simulink model "Non_linear_damper"  (R2023b)
settings: Solver=VariableStepAuto  StartTime=0.0  StopTime=10.0  RelTol=1e-3
values from neighbouring files (symbols this model uses):
  Ks = params.Ks    [Non-_inear_damper.m]    (also in Non_linear_damper.m; Non_linear_damper_v2.m; Sim1_stable.m = 100; Simulation1.m = 100)
  Kt = params.Kt    [Non-_inear_damper.m]    (also in Non_linear_damper.m; Non_linear_damper_v2.m; Sim1_stable.m = 1000; Simulation1.m = 1000)
  ms = params.ms    [Non-_inear_damper.m]    (also in Non_linear_damper.m; Non_linear_damper_v2.m; Sim1_stable.m = 2.59027094234; Simulation1.m = 2.59027094234)
  mu = params.mu    [Non-_inear_damper.m]    (also in Non_linear_damper.m; Non_linear_damper_v2.m; Sim1_stable.m = 0.259027094234; Simulation1.m = 0.259027094234)
settings Model: Creator=youbotica  LastModifiedBy=youbotica

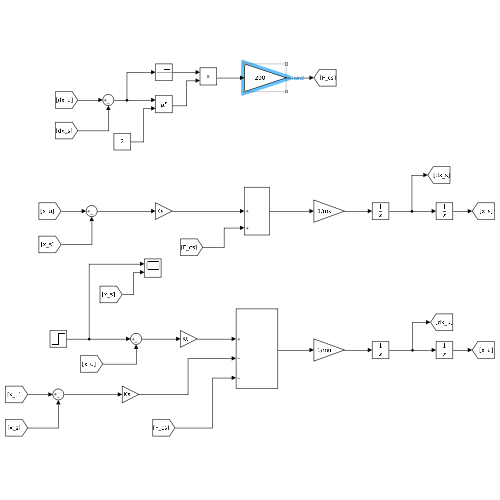
[thumbnail: Simulink's stored preview of the top-level diagram]
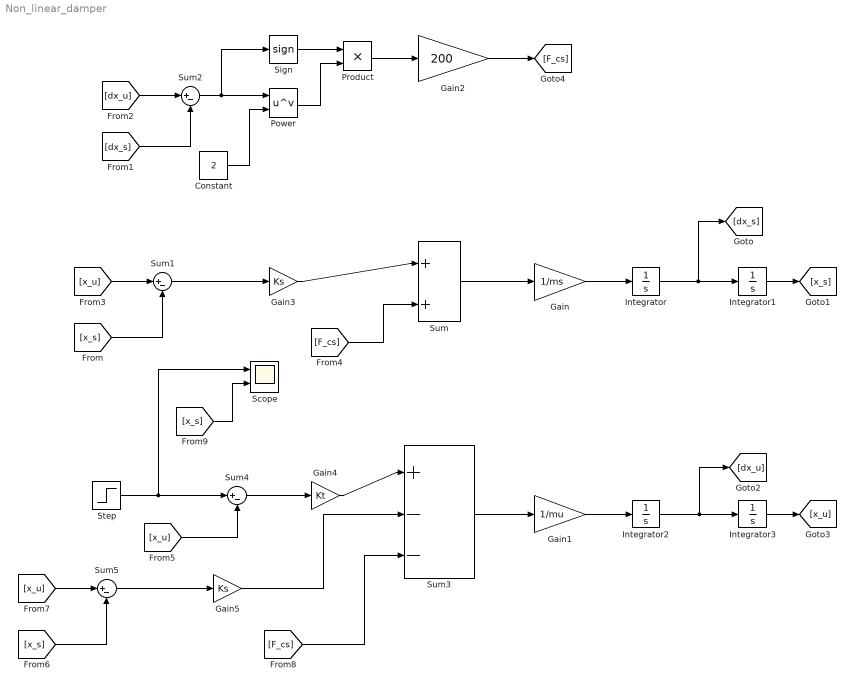
== system Non_linear_damper ==
  Constant : Constant  Value=2
  Gain : Gain  Gain=1/ms
  Gain1 : Gain  Gain=1/mu
  Gain2 : Gain  Gain=200
  Gain3 : Gain  Gain=Ks
  Gain4 : Gain  Gain=Kt
  Gain5 : Gain  Gain=Ks
  Integrator{,1..3} (4 alike) : Integrator
  Power : Math  Operator=pow
  Product : Product
  Scope : Scope  NumInputPorts=2
  Sign : Signum
  Step : Step  After=2  SampleTime=0
  Sum : Sum  Inputs=|++
  Sum{1..2,4..5} (4 alike) : Sum  Inputs=|+-
  Sum3 : Sum  Inputs=|+--
  wires:
  Integrator/1 -> [dx_s], Integrator1/1
  Integrator2/1 -> [dx_u], Integrator3/1
  Gain1/1 -> Integrator2/1
  Gain/1 -> Integrator/1
  Sum/1 -> Gain/1
  Integrator1/1 -> [x_s]
  Integrator3/1 -> [x_u]
  [x_s] -> Sum1/2
  [x_u] -> Sum1/1
  Sum1/1 -> Gain3/1
  Gain3/1 -> Sum/1
  [dx_u] -> Sum2/1
  [dx_s] -> Sum2/2
  Sum2/1 -> Sign/1, Power/1
  Constant/1 -> Power/2
  Sign/1 -> Product/1
  Power/1 -> Product/2
  Product/1 -> Gain2/1
  Gain2/1 -> [F_cs]
  [F_cs] -> Sum/2
  Sum3/1 -> Gain1/1
  Gain4/1 -> Sum3/1
  Sum4/1 -> Gain4/1
  [x_u] -> Sum4/2
  Step/1 -> Scope/1, Sum4/1
  Sum5/1 -> Gain5/1
  [x_u] -> Sum5/1
  [x_s] -> Sum5/2
  Gain5/1 -> Sum3/2
  [F_cs] -> Sum3/3
  [x_s] -> Scope/2
